simulink model "IMU_hand_linked"  (R2021b)
settings: Solver=ode1  StartTime=0.0  StopTime=300  FixedStep=.002  RelTol=1e-3  EnableMultiTasking=on
undefined symbols (not defined in the file): deg, s
libraries: qbmove_library x2, CP_library x1, QB_pacer_lib x1
settings Model: Creator=laurentio  LastModifiedBy=Mattia
settings SolverCC: AlgebraicLoopSolver=TrustRegion
settings DataIOCC: LimitDataPoints=on  SaveFormat=Array  ReturnWorkspaceOutputs=off
settings OptimizationCC: LifeSpan=inf
settings DebuggingCC: UnderspecifiedInitializationDetection=Classic  MergeDetectMultiDrivingBlocksExec=none  SolverPrmCheckMsg=warning  AllowSymbolicDim=off  StateNameClashWarn=warning  SFUnexpectedBacktrackingDiag=warning  SFNoUnconditionalDefaultTransitionDiag=warning  SFExecutionAtInitializationDiag=none  SFMachineParentedDataDiag=warning  ArithmeticOperatorsInVariantConditions=warning
settings HardwareCC: ProdBitPerPointer=32  ProdBitPerSizeT=32  ProdBitPerPtrDiffT=32  ProdLargestAtomicFloat=None  ProdIntDivRoundTo=Undefined  ProdEndianess=Unspecified  ProdWordSize=32  ProdHWDeviceType=32-bit Generic
settings ModelReferenceCC: PropagateSignalLabelsOutOfModel=off
settings SFSimCC: SimUseLocalCustomCode=off  CustomCodeUndefinedFunction=UseInterfaceOnly
settings RTWCC: RTWUseLocalCustomCode=off
settings CodeAppCC: StateflowObjectComments=on
settings GRTTargetCC: TargetLangStandard=C89/C90 (ANSI)
settings ConfigComp: CovMetricSettings=dw  CovSaveCumulativeToWorkspaceVar=on  CovSaveSingleToWorkspaceVar=on  CovExternalEMLEnable=off  CovSFcnEnable=off

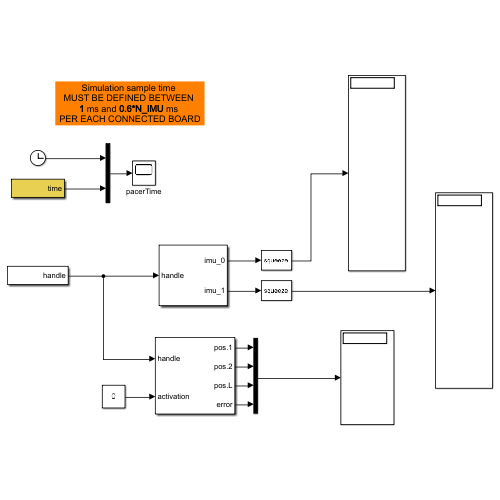
[thumbnail: Simulink's stored preview of the top-level diagram]
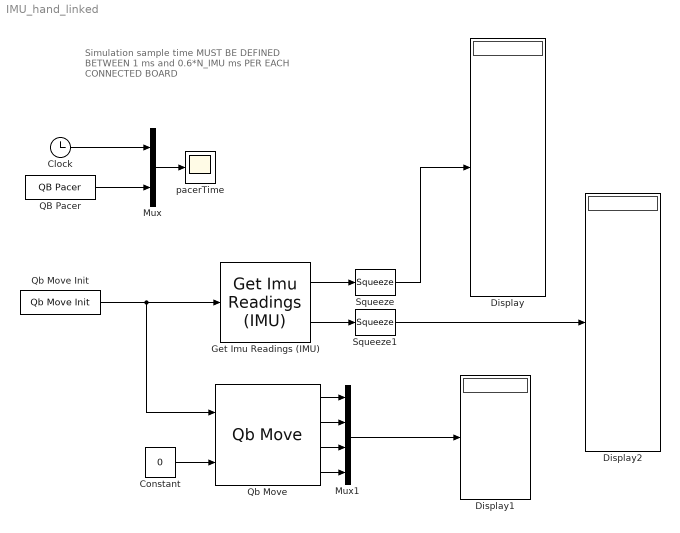
== system IMU_hand_linked ==
  note: Simulation sample time
      | MUST BE DEFINED BETWEEN
      | 1 ms and 0.6*N_IMU ms
      | PER EACH CONNECTED BOARD
  Clock : Clock
  Constant : Constant  Value=0
  Display : Display
  Display1 : Display
  Display2 : Display
  Get Imu Readings (IMU) : CP_library/Get Imu Readings (IMU)  ID=1  N_IMU=2  DAISY_CHAINING=off  ACC_UNITY=G  GYRO_UNITY=deg/s  MAG_UNITY=uT
      settings: SourceProductName=Centro Piaggio Library
  Mux : Mux  Inputs=2
  Mux1 : Mux
  QB Pacer : QB_pacer_lib/QB Pacer  simTimePerRealTime=1
      settings: SourceProductName=QB Pacer
  Qb Move : qbmove_library/Qb Move  ID=2  ACTIVE_COMM_DIRECTIONS=Rx  CONTROL_MODE=Prime Movers Positions  DAISY_CHAINING=off  MAX_ANG=0  SW_LIMIT=inf  OFFSET=0  ACTIVATE=off  WDT=0.0  UNIT=Degrees
      settings: SourceProductName=Qb Move Library
  Qb Move Init : qbmove_library/Qb Move Init  NUMBER_OF_COM='COM1'  BAUD_RATE_COM=2000000
      settings: SourceProductName=Qb Move Library
  Squeeze : Squeeze
  Squeeze1 : Squeeze
  pacerTime : Scope
  wires:
  QB Pacer/1 -> Mux/2
  Clock/1 -> Mux/1
  Qb Move Init/1 -> Get Imu Readings (IMU)/1, Qb Move/1
  Mux/1 -> pacerTime/1
  Get Imu Readings (IMU)/1 -> Squeeze/1
  Get Imu Readings (IMU)/2 -> Squeeze1/1
  Qb Move/1 -> Mux1/1
  Qb Move/2 -> Mux1/2
  Qb Move/3 -> Mux1/3
  Qb Move/4 -> Mux1/4
  Mux1/1 -> Display1/1
  Constant/1 -> Qb Move/2
  Squeeze/1 -> Display/1
  Squeeze1/1 -> Display2/1
